simulink model "PathVisualization"  (R2020a)
settings: Solver=VariableStepAuto  StartTime=0.0  StopTime=67  RelTol=1e-3
libraries: vrlib x1
settings Model: Creator=Abdul Hannan  LastModifiedBy=Abdul Hannan

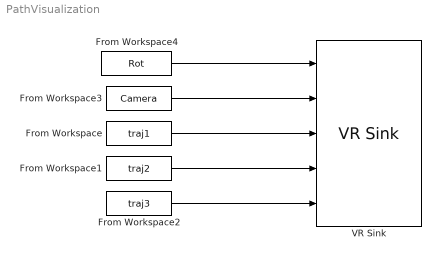
== system PathVisualization ==
  From Workspace : FromWorkspace  VariableName=traj1  OutDataTypeStr=double
  From Workspace1 : FromWorkspace  VariableName=traj2  OutDataTypeStr=double
  From Workspace2 : FromWorkspace  VariableName=traj3  OutDataTypeStr=double
  From Workspace3 : FromWorkspace  VariableName=Camera
  From Workspace4 : FromWorkspace  VariableName=Rot
  VR Sink : vrlib/VR Sink  InstantiateOnLoad=on  SampleTime=0.02  ViewEnable=on  RemoteChange=off  RemoteView=off  FieldsWritten=View.rotation.4.1.1.double#View.translation.3.1.1.double#Drone1.translation.3.1.1.double#Drone2.translation.3.1.1.double#Drone3.translation.3.1.1.double  WorldFileName=World-Model\Disaster_Prob.x3d  AutoView=on  VideoDimensions=[]  AllowVariableSize=off
  wires:
  From Workspace/1 -> VR Sink/3
  From Workspace1/1 -> VR Sink/4
  From Workspace2/1 -> VR Sink/5
  From Workspace3/1 -> VR Sink/2
  From Workspace4/1 -> VR Sink/1
